simulink model "bus_roadtest_v3"  (R2018a)
settings: Solver=ode3  StartTime=0.0  StopTime=inf  FixedStep=0.01  RelTol=1e-3  EnableMultiTasking=on
PostLoadFcn:
  | , if any(exist('dsrtsu_mdlpostloadfcn', 'file') == [2, 3, 6]), try dsrtsu_mdlpostloadfcn('Execute', bdroot); catch fprintf('Error in PostLoadFcn (dsrtsu_mdlpostloadfcn) for model "%s":\n %s\n', bdroot, lasterr); end, end,
InitFcn:
  | bus_roadtest_v3_initial
values from neighbouring files (symbols this model uses):
  ay_max = 2    [Ini.m]
  delta_t = 0.01    [Ini.m]
  end_left_pass = 1    [Ini.m]
  end_right_pass = 0    [Ini.m]
  finish_node_id = length(Map_data(:,1))    [Ini.m]
  forward_length = 15    [Ini.m]
  gamma = sqrt(N_xaug+lambda)    [bus_roadtest_v3_initial.m]
  k_safe = 1    [Ini.m]
  nodes = nodes(1:index_node,:)    [Ini.m]
  rmin = 10    [Ini.m]
  segments = zeros(length(xy_ends_Pos(:,1)),3)    [Ini.m]
  start_node_id = 1    [Ini.m]
  Ts = 0.01    [bus_roadtest_v3_initial.m]
  Veh_CG = [0.5, 0.2]    [Ini.m]
  Veh_size = [1.99986,6.09558]    [Ini.m]
  vmax = 6    [Ini.m]
  weight = [weight_0,weight_0_cov,weight_i]    [bus_roadtest_v3_initial.m]
undefined symbols (not defined in the file or in its folder): Brake_table, DiscIntNeverNeededParam, Map_data, R, REF_GPS_RFS, Steer_gain_table, T
libraries: rtican x71, simulink x26, rti1401lib_adc_type4 x8, rti1401lib_dio_type4 x1
(part 17 of 18)

== matlab function bus_roadtest_v3/Target_planner/DynamicPathPlanning ==
  data: Path_flag input; Static_Path_0 input size=size(Map_data); Path_final output; XP_final output; YP_final output; Forward_Static_Path_id input size=length(nodes(:,1)); End_x input; End_y input; Vehicle_state input; seg_Curvature input; path_length input; end_right_pass input; end_left_pass input; Veh_CG input; Veh_size input; OB_num input; OBXY input; rmin input; Veh_Velocity input; delta_t input; ay_max input; vmax input; k_safe input; w_off input; LastPath_in input; v_final output; end_point_final output; end_curvature output; TargetXY output; Vehicle_Target_x output; Vehicle_Target_y output; vehicle_boundingbox_x output; vehicle_boundingbox_y output; J_out output; Jminind output; J_finalind output; L_path_final output; collision_check output
function [Path_final,XP_final,YP_final,v_final,end_point_final,end_curvature,TargetXY,Vehicle_Target_x,Vehicle_Target_y,vehicle_boundingbox_x,vehicle_boundingbox_y,J_out,Jminind,J_finalind,L_path_final,collision_check] = DynamicPathPlanning(Path_flag,Static_Path_0,Forward_Static_Path_id,End_x,End_y,Vehicle_state,seg_Curvature,path_length,end_right_pass,end_left_pass,Veh_CG,Veh_size,OB_num,OBXY,rmin,Veh_Velocity,delta_t,ay_max,vmax,k_safe,w_off,LastPath_in)

persistent LastPath
if isempty(LastPath)
    LastPath = zeros(11,2);
else
    LastPath = LastPath_in;
end

x_vehicle = Vehicle_state(1,1); %vehicle global coordinate
y_vehicle = Vehicle_state(2,1);
start_heading = Vehicle_state(3,1);

end_heading_0 = Static_Path_0(Forward_Static_Path_id(end) == Static_Path_0(:,1),8)*pi/180;
end_curvature_0 = Static_Path_0(Forward_Static_Path_id(end) == Static_Path_0(:,1),14);
end_seg_LaneWidth_0 = Static_Path_0(Forward_Static_Path_id(end) == Static_Path_0(:,1),11);
end_heading = end_heading_0(1);
end_curvature = end_curvature_0(1);
end_seg_LaneWidth = end_seg_LaneWidth_0(1);

delta_offset = end_seg_LaneWidth/4;
offset_1 = delta_offset*1;
offset_2 = delta_offset*2;
offset_3 = delta_offset*3;
offset_4 = delta_offset*4;
offset_5 = delta_offset*5;
offset_6 = delta_offset*6;
offset = [offset_6 offset_5 offset_4 offset_3 offset_2 offset_1 0 offset_1 offset_2 offset_3 offset_4 offset_5 offset_6];

x_endpoint1 = End_x + offset_6*cos(end_heading+pi/2);
y_endpoint1 = End_y + offset_6*sin(end_heading+pi/2);
x_endpoint2 = End_x + offset_5*cos(end_heading+pi/2);
y_endpoint2 = End_y + offset_5*sin(end_heading+pi/2);
x_endpoint3 = End_x + offset_4*cos(end_heading+pi/2);
y_endpoint3 = End_y + offset_4*sin(end_heading+pi/2);
x_endpoint4 = End_x + offset_3*cos(end_heading+pi/2);
y_endpoint4 = End_y + offset_3*sin(end_heading+pi/2);
x_endpoint5 = End_x + offset_2*cos(end_heading+pi/2);
y_endpoint5 = End_y + offset_2*sin(end_heading+pi/2);
x_endpoint6 = End_x + offset_1*cos(end_heading+pi/2);
y_endpoint6 = End_y + offset_1*sin(end_heading+pi/2);
x_endpoint7 = End_x;
y_endpoint7 = End_y;
x_endpoint8 = End_x + offset_1*cos(end_heading-pi/2);
y_endpoint8 = End_y + offset_1*sin(end_heading-pi/2);
x_endpoint9 = End_x + offset_2*cos(end_heading-pi/2);
y_endpoint9 = End_y + offset_2*sin(end_heading-pi/2);
x_endpoint10 = End_x + offset_3*cos(end_heading-pi/2);
y_endpoint10 = End_y + offset_3*sin(end_heading-pi/2);
x_endpoint11 = End_x + offset_4*cos(end_heading-pi/2);
y_endpoint11 = End_y + offset_4*sin(end_heading-pi/2);
x_endpoint12 = End_x + offset_5*cos(end_heading-pi/2);
y_endpoint12 = End_y + offset_5*sin(end_heading-pi/2);
x_endpoint13 = End_x + offset_6*cos(end_heading-pi/2);
y_endpoint13 = End_y + offset_6*sin(end_heading-pi/2);

%% Candidate paths generation
[X1,Y1,XP1,YP1,K1,K_11,L_path1] = G2splines(x_vehicle,y_vehicle,start_heading,seg_Curvature,x_endpoint1,y_endpoint1,end_heading,end_curvature,path_length);
[X2,Y2,XP2,YP2,K2,K_12,L_path2] = G2splines(x_vehicle,y_vehicle,start_heading,seg_Curvature,x_endpoint2,y_endpoint2,end_heading,end_curvature,path_length);
[X3,Y3,XP3,YP3,K3,K_13,L_path3] = G2splines(x_vehicle,y_vehicle,start_heading,seg_Curvature,x_endpoint3,y_endpoint3,end_heading,end_curvature,path_length);
[X4,Y4,XP4,YP4,K4,K_14,L_path4] = G2splines(x_vehicle,y_vehicle,start_heading,seg_Curvature,x_endpoint4,y_endpoint4,end_heading,end_curvature,path_length);
[X5,Y5,XP5,YP5,K5,K_15,L_path5] = G2splines(x_vehicle,y_vehicle,start_heading,seg_Curvature,x_endpoint5,y_endpoint5,end_heading,end_curvature,path_length);
[X6,Y6,XP6,YP6,K6,K_16,L_path6] = G2splines(x_vehicle,y_vehicle,start_heading,seg_Curvature,x_endpoint6,y_endpoint6,end_heading,end_curvature,path_length);
[X7,Y7,XP7,YP7,K7,K_17,L_path7] = G2splines(x_vehicle,y_vehicle,start_heading,seg_Curvature,x_endpoint7,y_endpoint7,end_heading,end_curvature,path_length);
[X8,Y8,XP8,YP8,K8,K_18,L_path8] = G2splines(x_vehicle,y_vehicle,start_heading,seg_Curvature,x_endpoint8,y_endpoint8,end_heading,end_curvature,path_length);
[X9,Y9,XP9,YP9,K9,K_19,L_path9] = G2splines(x_vehicle,y_vehicle,start_heading,seg_Curvature,x_endpoint9,y_endpoint9,end_heading,end_curvature,path_length);
[X10,Y10,XP10,YP10,K10,K_110,L_path10] = G2splines(x_vehicle,y_vehicle,start_heading,seg_Curvature,x_endpoint10,y_endpoint10,end_heading,end_curvature,path_length);
[X11,Y11,XP11,YP11,K11,K_111,L_path11] = G2splines(x_vehicle,y_vehicle,start_heading,seg_Curvature,x_endpoint11,y_endpoint11,end_heading,end_curvature,path_length);
[X12,Y12,XP12,YP12,K12,K_112,L_path12] = G2splines(x_vehicle,y_vehicle,start_heading,seg_Curvature,x_endpoint12,y_endpoint12,end_heading,end_curvature,path_length);
[X13,Y13,XP13,YP13,K13,K_113,L_path13] = G2splines(x_vehicle,y_vehicle,start_heading,seg_Curvature,x_endpoint13,y_endpoint13,end_heading,end_curvature,path_length);

X = [X1 X2 X3 X4 X5 X6 X7 X8 X9 X10 X11 X12 X13];
Y = [Y1 Y2 Y3 Y4 Y5 Y6 Y7 Y8 Y9 Y10 Y11 Y12 Y13];
XP = [XP1 XP2 XP3 XP4 XP5 XP6 XP7 XP8 XP9 XP10 XP11 XP12 XP13];
YP = [YP1 YP2 YP3 YP4 YP5 YP6 YP7 YP8 YP9 YP10 YP11 YP12 YP13];
K = [K1 K2 K3 K4 K5 K6 K7 K8 K9 K10 K11 K12 K13];
K_1 = [K_11 K_12 K_13 K_14 K_15 K_16 K_17 K_18 K_19 K_110 K_111 K_112 K_113];
L_path = [L_path1 L_path2 L_path3 L_path4 L_path5 L_path6 L_path7 L_path8 L_path9 L_path10 L_path11 L_path12 L_path13];
xy_end_point = [x_endpoint1,x_endpoint2,x_endpoint3,x_endpoint4,x_endpoint5,x_endpoint6,x_endpoint7,x_endpoint8,x_endpoint9,x_endpoint10,x_endpoint11,x_endpoint12,x_endpoint13;y_endpoint1,y_endpoint2,y_endpoint3,y_endpoint4,y_endpoint5,y_endpoint6,y_endpoint7,y_endpoint8,y_endpoint9,y_endpoint10,y_endpoint11,y_endpoint12,y_endpoint13];

%% Collision check
Path_col = zeros(4,length(X(1,:))); %[Collision T/F ; Path collision ind ; OB num ; Lane collision T/F]
% Lane collision check
if end_right_pass == 0
    Path_col(4,9:13) = 1;
end
if end_left_pass == 0
    Path_col(4,1:5) = 1;
end

% Obstacle collision check
% Obstacle enlarge
OBXY_EL = OBXY;
OB_enlargescale = 0.3;
OB_enlargescale_behind = 0.3;
for m = 1 : OB_num
    OBXY_m = OBXY(2*m-1:2*m,1:4);
    OBXY_EL(2*m-1:2*m,1) = [OBXY_m(1,1) + (OBXY_m(1,1)-OBXY_m(1,2))*OB_enlargescale + (OBXY_m(1,1)-OBXY_m(1,4))*OB_enlargescale ; OBXY_m(2,1) + (OBXY_m(2,1)-OBXY_m(2,2))*OB_enlargescale + (OBXY_m(2,1)-OBXY_m(2,4))*OB_enlargescale];
    OBXY_EL(2*m-1:2*m,2) = [OBXY_m(1,2) + (OBXY_m(1,2)-OBXY_m(1,1))*OB_enlargescale + (OBXY_m(1,2)-OBXY_m(1,3))*OB_enlargescale ; OBXY_m(2,2) + (OBXY_m(2,2)-OBXY_m(2,1))*OB_enlargescale + (OBXY_m(2,2)-OBXY_m(2,3))*OB_enlargescale];
    OBXY_EL(2*m-1:2*m,3) = [OBXY_m(1,3) + (OBXY_m(1,3)-OBXY_m(1,4))*OB_enlargescale + (OBXY_m(1,3)-OBXY_m(1,2))*OB_enlargescale_behind ; OBXY_m(2,3) + (OBXY_m(2,3)-OBXY_m(2,4))*OB_enlargescale + (OBXY_m(2,3)-OBXY_m(2,2))*OB_enlargescale_behind];
    OBXY_EL(2*m-1:2*m,4) = [OBXY_m(1,4) + (OBXY_m(1,4)-OBXY_m(1,3))*OB_enlargescale + (OBXY_m(1,4)-OBXY_m(1,1))*OB_enlargescale_behind ; OBXY_m(2,4) + (OBXY_m(2,4)-OBXY_m(2,3))*OB_enlargescale + (OBXY_m(2,4)-OBXY_m(2,1))*OB_enlargescale_behind];
end
% 計算每條線的每個sample點的單位向量及法向量
X_1 = X(1:end-1,:);
X_2 = X(2:end,:);
X_diff_0 = X_2 - X_1;
X_diff = [X_diff_0(:,:);X_diff_0(end,:)];
Y_1 = Y(1:end-1,:);
Y_2 = Y(2:end,:);
Y_diff_0 = Y_2 - Y_1;
Y_diff = [Y_diff_0(:,:);Y_diff_0(end,:)];
XY_difflen = (X_diff.^2 + Y_diff.^2).^0.5;
X_UV = X_diff./XY_difflen; %X方向單位向量(Unit Vector)
Y_UV = Y_diff./XY_difflen; %Y方向單位向量(Unit Vector)
X_NV = -Y_UV; %X方向單位法向量(Normal Vector)
Y_NV = X_UV; %Y方向單位法向量(Normal Vector)
% 計算veh四個角位置
Path_vehFLX = X + Veh_CG(1)*Veh_size(1).*X_NV + Veh_CG(2)*Veh_size(2).*X_UV;
Path_vehFLY = Y + Veh_CG(1)*Veh_size(1).*Y_NV + Veh_CG(2)*Veh_size(2).*Y_UV;
Path_vehFRX = X - (1-Veh_CG(1))*Veh_size(1).*X_NV + Veh_CG(2)*Veh_size(2).*X_UV;
Path_vehFRY = Y - (1-Veh_CG(1))*Veh_size(1).*Y_NV + Veh_CG(2)*Veh_size(2).*Y_UV;
Path_vehRLX = X + Veh_CG(1)*Veh_size(1).*X_NV - (1-Veh_CG(2))*Veh_size(2).*X_UV;
Path_vehRLY = Y + Veh_CG(1)*Veh_size(1).*Y_NV - (1-Veh_CG(2))*Veh_size(2).*Y_UV;
Path_vehRRX = X - (1-Veh_CG(1))*Veh_size(1).*X_NV - (1-Veh_CG(2))*Veh_size(2).*X_UV;
Path_vehRRY = Y - (1-Veh_CG(1))*Veh_size(1).*Y_NV - (1-Veh_CG(2))*Veh_size(2).*Y_UV;
% project to normal vector
for i = 1 : length(Path_vehFLX(1,:))
    Path_col(1,i) = 0;
    if Path_col(4,i) == 1
        continue;
    else
        for j = 1 : length(Path_vehFLX(:,1))
            Path_vehvol = [Path_vehFLX(j,i),Path_vehFRX(j,i),Path_vehRLX(j,i),Path_vehRRX(j,i);Path_vehFLY(j,i),Path_vehFRY(j,i),Path_vehRLY(j,i),Path_vehRRY(j,i)];
            for k = 1 : OB_num
                OBXY_k = OBXY_EL(2*k-1:2*k,1:4);
                % obstcale normal vector
                OBnormal1 = [-(OBXY_k(2,2)-OBXY_k(2,1)),(OBXY_k(1,2)-OBXY_k(1,1))]./sqrt((OBXY_k(1,2)-OBXY_k(1,1))^2 + (OBXY_k(1,2)-OBXY_k(1,1))^2);
                OBnormal2 = [-(OBXY_k(2,3)-OBXY_k(2,2)),(OBXY_k(1,3)-OBXY_k(1,2))]./sqrt((OBXY_k(2,3)-OBXY_k(2,2))^2 + (OBXY_k(1,3)-OBXY_k(1,2))^2);
                proj_veh = [OBnormal1;OBnormal2;[X_UV(j,i),Y_UV(j,i)];[X_NV(j,i),Y_NV(j,i)]] * Path_vehvol;
                proj_ob = [OBnormal1;OBnormal2;[X_UV(j,i),Y_UV(j,i)];[X_NV(j,i),Y_NV(j,i)]] * OBXY_k;
                minmax_veh = [min(proj_veh,[],2),max(proj_veh,[],2)];
                minmax_obj = [min(proj_ob,[],2),max(proj_ob,[],2)];

                % check if vehicle collide with specify object at the chosen point
                for r = 1:4
                    if (minmax_veh(r,1)>minmax_obj(r,2) || minmax_veh(r,2)<minmax_obj(r,1))
                        Path_col(1,i) = 0;
                        break;      % ends SAT with a object
                    end
                    Path_col(1,i) = 1;
                end
                % Collision happens and ends the object checking process
                if Path_col(1,i) == 1
                    Path_col(3,i) = k;
                    break;         % ends all object checking
                end
            end
            % Collision happens and ends the point checking process
            if Path_col(1,i) == 1
                Path_col(2,i) = j;
                break;          % ends point checking
            end
        end
    end
end
% Gaussian concolution
Cobs_0 = Path_col(1,:);
Cobs = Cobs_0;
sigma = std(Cobs_0(1,:));
delta_q = 1;
Path_index = 1:1:length(Cobs_0(1,:));
if sigma ~= 0
    for i = 1 : length(Cobs_0(1,:))
        Path_index_i = i*ones(size(Path_index));
        Path_index_diff = Path_index_i - Path_index;
        g = exp(-(delta_q.*Path_index_diff).^2./(2*sigma^2))./(sqrt(2*pi)*sigma);
        Cobs(1,i) = sum(Cobs_0(1,:).*g);
        if i == 1 && Cobs_0(1,1) == 1
            Cobs(1,i) = Cobs(1,i) + exp(-(delta_q.*1).^2./(2*sigma^2))./(sqrt(2*pi)*sigma);
        elseif i == length(Cobs_0(1,:)) && Cobs_0(1,end) == 1
            Cobs(1,i) = Cobs(1,i) + exp(-(delta_q.*1).^2./(2*sigma^2))./(sqrt(2*pi)*sigma);
        else
            Cobs(1,i) = Cobs(1,i);
        end
    end
    if max(Cobs(1,:)) ~= 1
        Cobs(1,:) = Cobs(1,:)./max(Cobs(1,:));
    end
end
% Cobs1 = Cobs;
% if sigma ~= 0
%     Cobs1(1,:) = imgaussfilt(Path_col(1,:),sigma); %matlab內建gaussian concolution
% end
Clane_0 = Path_col(4,:);
Clane = Clane_0;
sigma = std(Clane_0(1,:));
delta_q = 1;
Path_index = 1:1:length(Clane_0(1,:));
if sigma ~= 0
    for i = 1 : length(Clane_0(1,:))
        Path_index_i = i*ones(size(Path_index));
        Path_index_diff = Path_index_i - Path_index;
        g = exp(-(delta_q.*Path_index_diff).^2./(2*sigma^2))./(sqrt(2*pi)*sigma);
        Clane(1,i) = sum(Clane_0(1,:).*g);
        if i == 1 && Clane_0(1,1) == 1
            Clane(1,i) = Clane(1,i) + exp(-(delta_q.*1).^2./(2*sigma^2))./(sqrt(2*pi)*sigma);
        elseif i == length(Clane_0(1,:)) && Clane_0(1,end) == 1
            Clane(1,i) = Clane(1,i) + exp(-(delta_q.*1).^2./(2*sigma^2))./(sqrt(2*pi)*sigma);
        else
            Clane(1,i) = Clane(1,i);
        end
    end
    if max(Clane(1,:)) ~= 1
        Clane(1,:) = Clane(1,:)./max(Clane(1,:));
    end
end
%% Consistency
Cc_0 = zeros(1,length(X(1,:)));
% current vehicle postion to last path
[~,Lastpath_si] = min(sqrt((LastPath(:,1) - x_vehicle).^2 + (LastPath(:,2) - y_vehicle).^2));
LastPath_overlap = LastPath(Lastpath_si:end,:);

for k = 1 : length(X(1,:))
    % last end point to current paths
    [~,Pathk_ei] = min(sqrt((X(:,k) - LastPath(end,1)).^2 + (Y(:,k) - LastPath(end,2)).^2));
    Path_overlap = [X(1:Pathk_ei,k) Y(1:Pathk_ei,k)];
%     if length(LastPath_overlap(:,1)) >= length(Path_overlap(:,1))
%         Path_diff = length(LastPath_overlap(:,1)) - length(Path_overlap(:,1));
%         Path_dis = sqrt(sum(LastPath_overlap(1+Path_diff:end,:)-Path_overlap).^2);
%     else
%         Path_diff = length(Path_overlap(:,1)) - length(LastPath_overlap(:,1));
%         Path_dis = sqrt(sum(LastPath_overlap-Path_overlap(1+Path_diff:end,:)).^2);
%     end
    if length(LastPath_overlap(:,1)) >= length(Path_overlap(:,1))
        Path_diff = length(LastPath_overlap(:,1)) - length(Path_overlap(:,1));
%         Path_dis_xy = LastPath_overlap(1+Path_diff:end,:)-Path_overlap;
%         Path_dis = sqrt(Path_dis_xy(:,1).*Path_dis_xy(:,1) + Path_dis_xy(:,2).*Path_dis_xy(:,2));
        Path_dis_xy = (LastPath_overlap(1+Path_diff:end,:)-Path_overlap).^2;
        Path_dis = sqrt(sum(Path_dis_xy'));
        Path_dis = Path_dis';
    else
        Path_diff = length(Path_overlap(:,1)) - length(LastPath_overlap(:,1));
        Path_dis_xy = (LastPath_overlap(1:end,1:2) - Path_overlap(1:end-Path_diff,:)).^2;
        Path_dis = sqrt(sum(Path_dis_xy'));
        Path_dis = Path_dis';
    end
    if mod(length(Path_dis),2) == 0
        cons_simCoeff = 4*ones(1,length(Path_dis)-1);
    else
        cons_simCoeff = 4*ones(1,length(Path_dis));
    end
    cons_simCoeff([1,length(cons_simCoeff)]) = 1;
    cons_simCoeff(3:2:length(cons_simCoeff)-2) = 2;
    
    bframe_delta = L_path(k)/length(X(:,k));
    cons_overlapL = L_path(k)*length(Path_dis)/length(X(:,k));
    Path_sumdis = bframe_delta*(cons_simCoeff*Path_dis(1:length(cons_simCoeff))')/3;
    Cc_0(1,k) = Path_sumdis/cons_overlapL;
end

%% Cost function
% weighting
W = [0.5 1 1 w_off 30 10 30];
%   [ L   k  k_1 off obs c lane]

Cl = L_path./path_length;
Ck = (max(abs(K)).*rmin)./max(max(abs(K)).*rmin);
Ck_1 = (max(abs(K_1)).*rmin)./max(max(abs(K_1)).*rmin);
Coff = offset/max(offset);
Cobss = Cobs(1,:);%Path_col(1,:);%f*exp((-1/lamda).*d) + P;
if max(Cc_0) == 0
    Cc = Cc_0;
else
    Cc = Cc_0/max(Cc_0);
end
Clanes = Clane(1,:);%Path_col(1,:);%f*exp((-1/lamda).*d) + P;

% cost function
J = W(1).*Cl + W(2).*Ck + W(3).*Ck_1 + W(4).*Coff + W(5).*Cobss + W(6).*Cc + W(7).*Clanes;
[Jmin,Jminind] = min(J);

if Path_flag == 1
    J_finalind = Jminind;
else
    J_finalind = 7;
end

X_final = X(:,J_finalind);
Y_final = Y(:,J_finalind);
Path_final = [X_final,Y_final];
end_point_final = [xy_end_point(:,J_finalind);end_heading];
J_out = J';

%% Velocity decision
k_vehicle_max = 1/rmin;
if max(abs(K(J_finalind))) > k_vehicle_max
    k_max = k_vehicle_max;
else
    k_max = max(abs(K(J_finalind)));
end
v_k = sqrt(ay_max/k_max);
v_safe = (1-k_safe*Cobs(J_finalind)^2)*v_k;
if v_safe > vmax
    v_final = vmax; %(m/s)
else
    v_final = v_safe; %(m/s)
end

L_path_final = L_path(J_finalind);

%% Next Step Position
XP_final = XP(:,J_finalind);
YP_final = YP(:,J_finalind);
u_final_Target = (Veh_Velocity*1+3)/L_path(J_finalind);
x_target = XP_final(1) + XP_final(2)*u_final_Target + XP_final(3)*u_final_Target^2 + XP_final(4)*u_final_Target^3 + XP_final(5)*u_final_Target^4 + XP_final(6)*u_final_Target^5;
y_target = YP_final(1) + YP_final(2)*u_final_Target + YP_final(3)*u_final_Target^2 + YP_final(4)*u_final_Target^3 + YP_final(5)*u_final_Target^4 + YP_final(6)*u_final_Target^5;
TargetXY = [x_target;y_target];
vehicle_boundingbox_x = [Path_vehFLX(1,7);Path_vehFRX(1,7);Path_vehRRX(1,7);Path_vehRLX(1,7)];
vehicle_boundingbox_y = [Path_vehFLY(1,7);Path_vehFRY(1,7);Path_vehRRY(1,7);Path_vehRLY(1,7)];
%% vehicle target x y
heading = Vehicle_state(3,1);
rotate_ang = -heading;
Vehicle_Target = [cos(rotate_ang),-sin(rotate_ang);sin(rotate_ang),cos(rotate_ang)]*[x_target-x_vehicle;y_target-y_vehicle];
Vehicle_Target_x = Vehicle_Target(1);
Vehicle_Target_y = Vehicle_Target(2);

%%
collision_check = Cobs_0(J_finalind);
%% Function
function [X,Y,XP,YP,K,K_1,L_path] = G2splines(xa,ya,thetaa,ka,xb,yb,thetab,kb,path_length)
n1 = path_length; %optimization
n2 = n1;
n3 = 0; %越大切越大
n4 = -n3;

% n1 = path_length; %optimization
% n2 = n1;
% n3 = 50; %越大切越大
% n4 = -n3;

% n1 = path_length/3; %optimization
% n2 = n1;
% n3 = 50; %optimization
% n4 = -n3;

x0 = xa;
x1 = n1*cos(thetaa);
x2 = 0.5*(n3*cos(thetaa)-(n1^2)*ka*sin(thetaa));
x3 = 10*(xb-xa)-(6*n1+1.5*n3).*cos(thetaa)-(4*n2-0.5*n4).*cos(thetab)+1.5*(n1^2)*ka.*sin(thetaa)-0.5*(n2^2)*kb.*sin(thetab);
x4 = -15*(xb-xa)+(8*n1+1.5*n3).*cos(thetaa)+(7*n2-n4).*cos(thetab)-1.5*(n1^2)*ka.*sin(thetaa)+(n2^2)*kb.*sin(thetab);
x5 = 6*(xb-xa)-(3*n1+0.5*n3).*cos(thetaa)-(3*n2-0.5*n4).*cos(thetab)+0.5*(n1^2)*ka.*sin(thetaa)-0.5*(n2^2)*kb.*sin(thetab);
XP = [x0;x1;x2;x3;x4;x5];

y0 = ya;
y1 = n1*sin(thetaa);
y2 = 0.5*(n3*sin(thetaa)+(n1^2)*ka*cos(thetaa));
y3 = 10*(yb-ya)-(6*n1+1.5*n3).*sin(thetaa)-(4*n2-0.5*n4).*sin(thetab)-1.5*(n1^2)*ka.*cos(thetaa)+0.5*(n2^2)*kb.*cos(thetab);
y4 = -15*(yb-ya)+(8*n1+1.5*n3).*sin(thetaa)+(7*n2-n4).*sin(thetab)+1.5*(n1^2)*ka.*cos(thetaa)-(n2^2)*kb.*cos(thetab);
y5 = 6*(yb-ya)-(3*n1+0.5*n3).*sin(thetaa)-(3*n2-0.5*n4).*sin(thetab)-0.5.*(n1^2)*ka*cos(thetaa)+0.5.*(n2^2)*kb.*cos(thetab);
YP = [y0;y1;y2;y3;y4;y5];

u = 0 : 0.1 : 1;
u = u';
X = x0 + x1.*u + x2.*u.^2 + x3.*u.^3 + x4.*u.^4 + x5.*u.^5;
Y = y0 + y1.*u + y2.*u.^2 + y3.*u.^3 + y4.*u.^4 + y5.*u.^5;
X_1 = x1 + x2*2*u + x3*3*u.^2 + x4*4*u.^3 + x5*5*u.^4;
X_2 = x2*2 + x3*6*u + x4*12*u.^2 + x5*20*u.^3;
X_3 = x3*6 + x4*24*u + x5*60*u.^2;
Y_1 = y1 + y2*2*u + y3*3*u.^2 + y4*4*u.^3 + y5*5*u.^4;
Y_2 = y2*2 + y3*6*u + y4*12*u.^2 + y5*20*u.^3;
Y_3 = y3*6 + y4*24*u + y5*60*u.^2;
K = (X_1.*Y_2-X_2.*Y_1)./((X_1.^2+Y_1.^2).^1.5);
K_1 = ((X_1.^2+Y_1.^2).^1.5.*(X_2.*Y_2+X_1.*Y_3-X_3.*Y_1-X_2.*Y_2)-1.5.*(X_1.*Y_2-X_2.*Y_1).*(2.*X_1.*X_2+2.*Y_1.*Y_2).*((X_1.^2+Y_1.^2).^0.5))./((X_1.^2+Y_1.^2).^3);

% syms t
% XX_1 = x1 + x2*2*t + x3*3*t^2 + x4*4*t^3 + x5*5*t^4;
% YY_1 = y1 + y2*2*t + y3*3*t^2 + y4*4*t^3 + y5*5*t^4;
% f = (XX_1.^2+YY_1.^2).^0.5;
% L_path = double(int(f,t,0,1));
L_path = path_length;

== matlab function bus_roadtest_v3/Speed_profile/Auto & Check/Auto_start ==
  settings: updateMethod=DISCRETE
  data: Stop_Check input; Obj_detect input; AutoStart output; Emergency_stop input; AEB_count output; Drive_stop input; Drive_start input; AEBStatic output; AEBOn output; Static_flag input
function [AutoStart, AEB_count, AEBStatic, AEBOn] = fcn(Stop_Check, Obj_detect,Emergency_stop,Drive_stop,Drive_start, Static_flag)
persistent AEB_on counting AEB_static
if isempty(AEB_on)
    AEB_on = 0;
    counting = 0;
    AEB_static = 1;
end 
AutoStart = 0;

% if Obj_detect ==1 && Idle_flag ==0
if Obj_detect ==1
    AEB_on = 1;
end
if AEB_on==1 && Obj_detect==0 && Static_flag==1
    counting = counting+1;
elseif AEB_on==1 && Obj_detect==1
    counting = 0;
end
if counting>300 
    AEB_on = 0;
    counting = 0;
    AutoStart = 1;
end


% AEB_static will overwrite AutoStart
if Emergency_stop ==1 || Drive_stop ==1 ||  Stop_Check==1
    AEB_static = 1;
elseif Drive_start ==1
    AEB_static = 0;
    AEB_on = 0;
    counting = 0;
end
if AEB_static == 1
    AutoStart = 0;
end


% Output state
AEB_count = counting;
AEBStatic = AEB_static;
AEBOn = AEB_on;

== matlab function bus_roadtest_v3/Target_planner/DynamicPathPlanning1 ==
  data: Static_Path_0 input size=size(Map_data); Path_final output; XP_final output; YP_final output; Forward_Static_Path_id input size=length(nodes(:,1)); End_x input; End_y input; Jminind input; x_vehicle input; y_vehicle input; start_heading input; seg_Curvature input; path_length input; Veh_CG input; Veh_size input; OB_num input; OBXY input; collision_check output
function [Path_final,XP_final,YP_final,collision_check] = DynamicPathPlanning(Static_Path_0,Forward_Static_Path_id,End_x,End_y,Jminind,x_vehicle,y_vehicle,start_heading,seg_Curvature,path_length,Veh_CG,Veh_size,OB_num,OBXY)

% x_vehicle = Vehicle_state(1,1); %vehicle global coordinate
% y_vehicle = Vehicle_state(2,1);
% start_heading = Vehicle_state(3,1);

end_heading_0 = Static_Path_0(Forward_Static_Path_id(end) == Static_Path_0(:,1),8)*pi/180;
end_curvature_0 = Static_Path_0(Forward_Static_Path_id(end) == Static_Path_0(:,1),14);
end_seg_LaneWidth_0 = Static_Path_0(Forward_Static_Path_id(end) == Static_Path_0(:,1),11);
end_heading = end_heading_0(1);
end_curvature = end_curvature_0(1);
end_seg_LaneWidth = end_seg_LaneWidth_0(1);

delta_offset = end_seg_LaneWidth/4;
offset_1 = delta_offset*1;
offset_2 = delta_offset*2;
offset_3 = delta_offset*3;
offset_4 = delta_offset*4;
offset_5 = delta_offset*5;
offset_6 = delta_offset*6;
offset = [offset_6 offset_5 offset_4 offset_3 offset_2 offset_1 0 offset_1 offset_2 offset_3 offset_4 offset_5 offset_6];

offset_final = offset(Jminind);

if Jminind < 8
    x_endpoint = End_x + offset_final*cos(end_heading+pi/2);
    y_endpoint = End_y + offset_final*sin(end_heading+pi/2);
else
    x_endpoint = End_x + offset_final*cos(end_heading-pi/2);
    y_endpoint = End_y + offset_final*sin(end_heading-pi/2);
end

%% Candidate paths generation
[X_final,Y_final,XP_final,YP_final,K2,K_12,L_path2] = G2splines(x_vehicle,y_vehicle,start_heading,seg_Curvature,x_endpoint,y_endpoint,end_heading,end_curvature,path_length);
Path_final = [X_final,Y_final];

%% Collision check
Path_col = zeros(3,1); %[Collision T/F ; Path collision ind ; OB num ; Lane collision T/F]
% Obstacle collision check
% 計算每條線的每個sample點的單位向量及法向量
X_1 = X_final(1:end-1);
X_2 = X_final(2:end);
X_diff_0 = X_2 - X_1;
X_diff = [X_diff_0(:,:);X_diff_0(end,:)];
Y_1 = Y_final(1:end-1);
Y_2 = Y_final(2:end);
Y_diff_0 = Y_2 - Y_1;
Y_diff = [Y_diff_0(:,:);Y_diff_0(end,:)];
XY_difflen = (X_diff.^2 + Y_diff.^2).^0.5;
X_UV = X_diff./XY_difflen; %X方向單位向量(Unit Vector)
Y_UV = Y_diff./XY_difflen; %Y方向單位向量(Unit Vector)
X_NV = -Y_UV; %X方向單位法向量(Normal Vector)
Y_NV = X_UV; %Y方向單位法向量(Normal Vector)
% 計算veh四個角位置
Path_vehFLX = X_final + Veh_CG(1)*Veh_size(1).*X_NV + Veh_CG(2)*Veh_size(2).*X_UV;
Path_vehFLY = Y_final + Veh_CG(1)*Veh_size(1).*Y_NV + Veh_CG(2)*Veh_size(2).*Y_UV;
Path_vehFRX = X_final - (1-Veh_CG(1))*Veh_size(1).*X_NV + Veh_CG(2)*Veh_size(2).*X_UV;
Path_vehFRY = Y_final - (1-Veh_CG(1))*Veh_size(1).*Y_NV + Veh_CG(2)*Veh_size(2).*Y_UV;
Path_vehRLX = X_final + Veh_CG(1)*Veh_size(1).*X_NV - (1-Veh_CG(2))*Veh_size(2).*X_UV;
Path_vehRLY = Y_final + Veh_CG(1)*Veh_size(1).*Y_NV - (1-Veh_CG(2))*Veh_size(2).*Y_UV;
Path_vehRRX = X_final - (1-Veh_CG(1))*Veh_size(1).*X_NV - (1-Veh_CG(2))*Veh_size(2).*X_UV;
Path_vehRRY = Y_final - (1-Veh_CG(1))*Veh_size(1).*Y_NV - (1-Veh_CG(2))*Veh_size(2).*Y_UV;
% project to normal vector
Path_col(1) = 0;
for j = 1 : length(Path_vehFLX(:,1))
    Path_vehvol = [Path_vehFLX(j),Path_vehFRX(j),Path_vehRLX(j),Path_vehRRX(j);Path_vehFLY(j),Path_vehFRY(j),Path_vehRLY(j),Path_vehRRY(j)];
    for k = 1 : OB_num
        OBXY_k = OBXY(2*k-1:2*k,1:4);
        % obstcale normal vector
        OBnormal1 = [-(OBXY_k(2,2)-OBXY_k(2,1)),(OBXY_k(1,2)-OBXY_k(1,1))]./sqrt((OBXY_k(1,2)-OBXY_k(1,1))^2 + (OBXY_k(1,2)-OBXY_k(1,1))^2);
        OBnormal2 = [-(OBXY_k(2,3)-OBXY_k(2,2)),(OBXY_k(1,3)-OBXY_k(1,2))]./sqrt((OBXY_k(2,3)-OBXY_k(2,2))^2 + (OBXY_k(1,3)-OBXY_k(1,2))^2);
        proj_veh = [OBnormal1;OBnormal2;[X_UV(j),Y_UV(j)];[X_NV(j),Y_NV(j)]] * Path_vehvol;
        proj_ob = [OBnormal1;OBnormal2;[X_UV(j),Y_UV(j)];[X_NV(j),Y_NV(j)]] * OBXY_k;
        minmax_veh = [min(proj_veh,[],2),max(proj_veh,[],2)];
        minmax_obj = [min(proj_ob,[],2),max(proj_ob,[],2)];

        % check if vehicle collide with specify object at the chosen point
        for r = 1:4
            if (minmax_veh(r,1)>minmax_obj(r,2) || minmax_veh(r,2)<minmax_obj(r,1))
                Path_col(1) = 0;
                break;      % ends SAT with a object
            end
            Path_col(1) = 1;
        end
        % Collision happens and ends the object checking process
        if Path_col(1) == 1
            Path_col(3) = k;
            break;         % ends all object checking
        end
    end
    % Collision happens and ends the point checking process
    if Path_col(1) == 1
        Path_col(2) = j;
        break;          % ends point checking
    end
end
collision_check = Path_col(1);
%% Function
function [X,Y,XP,YP,K,K_1,L_path] = G2splines(xa,ya,thetaa,ka,xb,yb,thetab,kb,path_length)
n1 = path_length; %optimization
n2 = n1;
n3 = 0; %越大切越大
n4 = -n3;

% n1 = path_length; %optimization
% n2 = n1;
% n3 = 50; %越大切越大
% n4 = -n3;

% n1 = path_length/3; %optimization
% n2 = n1;
% n3 = 50; %optimization
% n4 = -n3;

x0 = xa;
x1 = n1*cos(thetaa);
x2 = 0.5*(n3*cos(thetaa)-(n1^2)*ka*sin(thetaa));
x3 = 10*(xb-xa)-(6*n1+1.5*n3).*cos(thetaa)-(4*n2-0.5*n4).*cos(thetab)+1.5*(n1^2)*ka.*sin(thetaa)-0.5*(n2^2)*kb.*sin(thetab);
x4 = -15*(xb-xa)+(8*n1+1.5*n3).*cos(thetaa)+(7*n2-n4).*cos(thetab)-1.5*(n1^2)*ka.*sin(thetaa)+(n2^2)*kb.*sin(thetab);
x5 = 6*(xb-xa)-(3*n1+0.5*n3).*cos(thetaa)-(3*n2-0.5*n4).*cos(thetab)+0.5*(n1^2)*ka.*sin(thetaa)-0.5*(n2^2)*kb.*sin(thetab);
XP = [x0;x1;x2;x3;x4;x5];

y0 = ya;
y1 = n1*sin(thetaa);
y2 = 0.5*(n3*sin(thetaa)+(n1^2)*ka*cos(thetaa));
y3 = 10*(yb-ya)-(6*n1+1.5*n3).*sin(thetaa)-(4*n2-0.5*n4).*sin(thetab)-1.5*(n1^2)*ka.*cos(thetaa)+0.5*(n2^2)*kb.*cos(thetab);
y4 = -15*(yb-ya)+(8*n1+1.5*n3).*sin(thetaa)+(7*n2-n4).*sin(thetab)+1.5*(n1^2)*ka.*cos(thetaa)-(n2^2)*kb.*cos(thetab);
y5 = 6*(yb-ya)-(3*n1+0.5*n3).*sin(thetaa)-(3*n2-0.5*n4).*sin(thetab)-0.5.*(n1^2)*ka*cos(thetaa)+0.5.*(n2^2)*kb.*cos(thetab);
YP = [y0;y1;y2;y3;y4;y5];

u = 0 : 0.1 : 1;
u = u';
X = x0 + x1.*u + x2.*u.^2 + x3.*u.^3 + x4.*u.^4 + x5.*u.^5;
Y = y0 + y1.*u + y2.*u.^2 + y3.*u.^3 + y4.*u.^4 + y5.*u.^5;
X_1 = x1 + x2*2*u + x3*3*u.^2 + x4*4*u.^3 + x5*5*u.^4;
X_2 = x2*2 + x3*6*u + x4*12*u.^2 + x5*20*u.^3;
X_3 = x3*6 + x4*24*u + x5*60*u.^2;
Y_1 = y1 + y2*2*u + y3*3*u.^2 + y4*4*u.^3 + y5*5*u.^4;
Y_2 = y2*2 + y3*6*u + y4*12*u.^2 + y5*20*u.^3;
Y_3 = y3*6 + y4*24*u + y5*60*u.^2;
K = (X_1.*Y_2-X_2.*Y_1)./((X_1.^2+Y_1.^2).^1.5);
K_1 = ((X_1.^2+Y_1.^2).^1.5.*(X_2.*Y_2+X_1.*Y_3-X_3.*Y_1-X_2.*Y_2)-1.5.*(X_1.*Y_2-X_2.*Y_1).*(2.*X_1.*X_2+2.*Y_1.*Y_2).*((X_1.^2+Y_1.^2).^0.5))./((X_1.^2+Y_1.^2).^3);

% syms t
% XX_1 = x1 + x2*2*t + x3*3*t^2 + x4*4*t^3 + x5*5*t^4;
% YY_1 = y1 + y2*2*t + y3*3*t^2 + y4*4*t^3 + y5*5*t^4;
% f = (XX_1.^2+YY_1.^2).^0.5;
% L_path = double(int(f,t,0,1));
L_path = path_length;

== matlab function bus_roadtest_v3/Flag_management/Fault detection/Fault detection(Control)/SLAM fault detection ==
  data: SLAM_FaultFlag input; y output; SLAM_MM_FaultFlag input
function y = fcn(SLAM_FaultFlag, SLAM_MM_FaultFlag)

y = max(SLAM_FaultFlag, SLAM_MM_FaultFlag);

== matlab function bus_roadtest_v3/Motion_controller/Longitudinal_control/Switching_module/MATLAB Function ==
  data: Speed_cmd input; T_resume output; Speed_bound input; upper_ratio input; lower_ratio input
function T_resume = T_shreshold(Speed_cmd,Speed_bound,upper_ratio,lower_ratio)

if Speed_cmd >= Speed_bound
    T_resume = upper_ratio;
else
    T_resume = lower_ratio + (Speed_cmd/Speed_bound)*(upper_ratio-lower_ratio);
end

== matlab function bus_roadtest_v3/Flag_management/State management/ BusStops ==
  settings: updateMethod=DISCRETE
  data: SLAM_X input; SLAM_Y input; Drive_start input; Stop_range input; BusStop_flag output; Stop_Distance output; Stop_cmd input; Stop_Mission input; Bus_state_forstop input; stop_acc output
function [BusStop_flag, Stop_Distance, stop_acc] = fcn(SLAM_X, SLAM_Y, Drive_start, Stop_range, Stop_cmd, Stop_Mission,Bus_state_forstop)

persistent BusStop_state NO_stop 
if isempty(BusStop_state)
    BusStop_state = 0;
    NO_stop = 0;
end 

% For SAND
% Stop_X = [  165.93, 1000000,    1000000,    1000000,    1000000,    1000000,    1000000,    1000000]; 
% Stop_Y = [  64.86,  1000000,    1000000,    1000000,     1000000,    1000000,    1000000,    1000000];


Stop_X = [  -12.192,    323.597,    600.409,    383.098,    33.200, 1000000, 1000000, 1000000]; 
Stop_Y = [  -114.466,   -282.300,   -194.395,   -45.546,    4.324,  1000000, 1000000, 1000000];
Stop_num = size(Stop_cmd,1);
for i=1:1:Stop_num
    if Stop_cmd(i)==0
        Stop_X(i) = 1000000;
        Stop_Y(i) = 1000000;
    end
end

if Stop_Mission ==99
    Stop_Distance = 1000;
else
    Stop_Distance = sqrt((SLAM_X-Stop_X(Stop_Mission))^2 + (SLAM_Y-Stop_Y(Stop_Mission))^2);
end

%%%%%%%%%%%%%%%%%%%%%%%%%%%%%%%%%%%%%%%%%%%%%%%%%%%%%%%%%%%%%%%%%%%%%%%%%%%
% Prevent Drive_start disable in checking zone
if Stop_Distance<5 && Drive_start==1
    NO_stop = 1;
end
if Stop_Distance>5.5 
    NO_stop = 0;
end

%%%%%%%%%%%%%%%%%%%%%%%%%%%%%%%%%%%%%%%%%%%%%%%%%%%%%%%%%%%%%%%%%%%%%%%%%%%
if Drive_start == 1
    BusStop_state = 0;
end
% Use distance for dicision
if Stop_Distance<Stop_range && Stop_Distance>(Stop_range-1) && NO_stop==0 && Bus_state_forstop==1
    BusStop_state = 1;
end
BusStop_flag = BusStop_state;

%%%%%%%%%%%%%%%%%%%%%%%%%%%%%%%%%%%%%%%%%%%%%%%%%%%%%%%%%%%%%%%%%%%%%%%%%%%

% Stop acc from accelerating in stop_zone
if Stop_Distance<30 && Bus_state_forstop==1 
    stop_acc = 1;
else
    stop_acc = 0;
end

== matlab function bus_roadtest_v3/Flag_management/State management/State_Management2 ==
  settings: updateMethod=DISCRETE
  data: Limit_range input; Zig_zag input; Fault_prime input; Fault_minor input; Idle_flag output; AEB_flag output; Digital_gate input; Static_flag input; Drive_start input; Auto_start input; Drive_stop input; BusStop_flag input; SlowMode_flag output; Emergency_stop input; Obj_detect output
function [Idle_flag, AEB_flag, SlowMode_flag, Obj_detect]= fcn(Limit_range,Zig_zag, Fault_prime, Fault_minor, Digital_gate, Static_flag, Drive_start, Auto_start, Drive_stop, BusStop_flag, Emergency_stop)

persistent Idle_state  AEB_state;
if isempty(Idle_state)
    Idle_state = 1;
    AEB_state = 0;
end 
%%%%%%%%%%%%%%%%%%%%%%%%%%%%%%%%%%%%%%%%%%%%%%%%%%%%%%%%%%%%%%%%%%%%%%%%%%%
%For Driving mode control
%Two buttons Drive_start & Drive_stop
% Only way to invalidate Idle_state, and disable AEB_state

% if (Drive_start == 1 || Auto_start == 1) && Static_flag == 1
if (Drive_start == 1 || Auto_start == 1) 
    Idle_state = 0;
    AEB_state= 0;
end
%%%%%%%%%%%%%%%%%%%%%%%%%%%%%%%%%%%%%%%%%%%%%%%%%%%%%%%%%%%%%%%%%%%%%%%%%%%
if Drive_stop == 1 
    Idle_state = 1;
end
%%%%%%%%%%%%%%%%%%%%%%%%%%%%%%%%%%%%%%%%%%%%%%%%%%%%%%%%%%%%%%%%%%%%%%%%%%%
if BusStop_flag == 1 
    Idle_state = 1;
end
%%%%%%%%%%%%%%%%%%%%%%%%%%%%%%%%%%%%%%%%%%%%%%%%%%%%%%%%%%%%%%%%%%%%%%%%%%%
%Fault Flag checking
if Fault_prime == 1
    Idle_state = 1;
end

%%%%%%%%%%%%%%%%%%%%%%%%%%%%%%%%%%%%%%%%%%%%%%%%%%%%%%%%%%%%%%%%%%%%%%%%%%%
% SlowMode_flag
%%%%%%%%%%%%%%%%%%%%%%%%%%%%%%%%%%%%%%%%%%%%%%%%%%%%%%%%%%%%%%%%%%%%%%%%%%%
if max([Zig_zag, Fault_minor]) ==1
    SlowMode_flag = 1;
else
    SlowMode_flag = 0;
end

%%%%%%%%%%%%%%%%%%%%%%%%%%%%%%%%%%%%%%%%%%%%%%%%%%%%%%%%%%%%%%%%%%%%%%%%%%%
% AEB_state
%%%%%%%%%%%%%%%%%%%%%%%%%%%%%%%%%%%%%%%%%%%%%%%%%%%%%%%%%%%%%%%%%%%%%%%%%%%
if    Emergency_stop == 1
    AEB_state = 1;
    Idle_state = 1;
end
%%%%%%%%%%%%%%%%%%%%%%%%%%%%%%%%%%%%%%%%%%%%%%%%%%%%%%%%%%%%%%%%%%%%%%%%%%%
Obj_detect = 0;
if  Digital_gate<Limit_range % For Demo (modified)
    AEB_state = 1;
    Idle_state = 1;
    Obj_detect = 1;
end
%%%%%%%%%%%%%%%%%%%%%%%%%%%%%%%%%%%%%%%%%%%%%%%%%%%%%%%%%%%%%%%%%%%%%%%%%%% 
Idle_flag = Idle_state;
AEB_flag = AEB_state;

== matlab function bus_roadtest_v3/Flag_management/State management/Map_defined_behavior ==
  data: ROS_near_segID input; Uturn_decel output; ROS_target_segID input; Uturn_gain output; Intersection_decel output; Uphill output; Uturn_gain_val output; Uturn_speed output
function [Uturn_decel,Uturn_gain,Intersection_decel,Uphill,Uturn_gain_val,Uturn_speed]  = Map_defined_behavior(ROS_near_segID,ROS_target_segID)

% ========== Initial parameters ==== %
persistent Gain_Uturn Decel_Uturn Decel_intersection Accel_Uphill
if isempty(Gain_Uturn)
    Gain_Uturn = 0;            % LKC gain should change to U-turn mode if Gain_Uturn == 1
    Decel_Uturn = 0;           % Speed_cmd should change to default speed for U-turn
    Decel_intersection = 0;    % Speed_cmd should change to default speed for passing intersection
    Accel_Uphill = 0;          % Speed_cmd should change to default speed for uphill section
end 

% ========== Map parameters =========%

% Map 1127
% intersection_seg = [24,38 ; 230,240];
% Uturn_seg =[4,19,20 ; 
%            43,60,18 ; 
%            75,84,20 ; 
%            97,108,20 ; 
%            109,126,18 ; 
%            155,165,20 ; 
%            168,180,20 ; 
%            203,215,20 ; 
%            219,232,20 ; 
%            285,297,20];
% Uturn_decel_seg = [4,19,7 ; 
%                    43,60,7 ; 
%                    75,84,7 ; 
%                    97,108,6 ; 
%                    109,126,5 ; 
%                    155,165,5 ; 
%                    168,180,5 ; 
%                    203,215,7 ; 
%                    219,232,10 ; 
%                    285,297,10];
% Uphill_seg = [96,104];

% Map 1127 & Rear axis control
intersection_seg = [24,38 ; 230,240];
Uturn_seg =[4,22,20 ; 
           43,65,20 ; 
           75,89,20 ; 
           97,109,20 ; 
           109,132,20 ; 
           155,168,20 ; 
           168,187,20 ; 
           203,216,20 ; 
           219,238,20 ; 
           285,302,20];
Uturn_decel_seg = [4,19,7 ; 
                   43,60,7 ; 
                   75,84,7 ; 
                   97,108,6 ; 
                   109,126,5 ; 
                   155,165,5 ; 
                   168,180,5 ; 
                   203,215,7 ; 
                   219,232,10 ; 
                   285,297,10];
Uphill_seg = [96,104];


% Map Tainan 0309
% intersection_seg = [2500,3000];
% Uturn_seg =[1,14,20 ; 
%            20,30,20 ; 
%            47,68,20 ; 
%            103,115,20 ; 
%            115,131,20 ; 
%            151,184,20 ; 
%            189,203,20 ; 
%            210,223,20 ; 
%            265,275,20 ; 
%            275,288,20 ;
%            327,341,20];
% Uturn_decel_seg = [1,14,5 ; 
%                    20,30,10 ; 
%                    47,68,10 ; 
%                    103,115,7 ; 
%                    115,131,7 ; 
%                    151,175,7 ; 
% %                    189,203,10 ; 
%                    210,223,7 ; 
%                    265,275,7 ; 
%                    275,288,7 ;
%                    327,341,5];
% Uphill_seg = [2000,3000];

% % Map Tainan 0312 (Bus stop)
% intersection_seg = [2500,3000];
% Uturn_seg =[19,30,30];
% Uturn_decel_seg = [2000,3000,10];
% Uphill_seg = [2000,3000];

% ========== Process ================%

for index_inter = 1:length(intersection_seg(:,1))
    if (ROS_target_segID >= intersection_seg(index_inter,1)) && (ROS_target_segID < intersection_seg(index_inter,2))
        Decel_intersection = 1;
        break;
    end
    Decel_intersection = 0;
end

for index_Uturn = 1:length(Uturn_seg(:,1))
    if (ROS_target_segID >= Uturn_seg(index_Uturn,1)) && (ROS_target_segID < Uturn_seg(index_Uturn,2))
        Gain_Uturn = 1;
        Uturn_gain_val = Uturn_seg(index_Uturn,3);
        break;
    end
    Gain_Uturn = 0;
    Uturn_gain_val = -1;
end

for index_Udecel = 1:length(Uturn_decel_seg(:,1))
    if (ROS_target_segID >= Uturn_decel_seg(index_Udecel,1)) && (ROS_target_segID < Uturn_decel_seg(index_Udecel,2))
        Decel_Uturn = 1;
        Uturn_speed = Uturn_decel_seg(index_Udecel,3);
        break;
    end
    Decel_Uturn = 0;
    Uturn_speed = -1;
end

for index_Uphill = 1:length(Uphill_seg(:,1))
    if (ROS_target_segID >= Uphill_seg(index_Uphill,1)) && (ROS_target_segID < Uphill_seg(index_Uphill,2))
        Accel_Uphill = 1;
        break;
    end
    Accel_Uphill = 0;
end

% ========== Flag output ============%

Uturn_gain = Gain_Uturn;
Uphill = Accel_Uphill;
if Uphill == 1
    Uturn_decel = 0;
    Intersection_decel = 0;
    Uturn_speed = -1;
else
    Uturn_decel = Decel_Uturn;
    Intersection_decel = Decel_intersection;
end

== matlab function bus_roadtest_v3/Flag_management/State management/TrafficLight ==
  settings: updateMethod=DISCRETE
  data: Light_Distance output; Light_flag output; Phase input; Light_acc output; SLAM_X input; SLAM_Y input; SLAM_seg_id_near input; Stop_Distance input; Drive_start input
function [Light_Distance, Light_flag, Light_acc] = fcn(Phase, SLAM_X, SLAM_Y,SLAM_seg_id_near, Stop_Distance, Drive_start)

%Stops & Light position on absolute coordinate
Light_X = [108.93, 118.31, 132.78];
Light_Y = [-9.39,  -20.71, -9.88];
Light_stop = [Light_X(3), Light_Y(3)];

% SAND
% Light_X = [  139.2,    160.79,    150.35,    133.28,    117.01, 136.09, 1000000, 1000000]; 
% Light_Y = [  88.74,   48.89,   19.88,   57.21,    92.42,  -11.87, 1000000, 1000000];
% if SLAM_seg_id_near>=114 && SLAM_seg_id_near<135
%     Light_stop = [Light_X(1), Light_Y(1)];
% elseif SLAM_seg_id_near>=135 && SLAM_seg_id_near<155
%     Light_stop = [Light_X(2), Light_Y(2)];
% elseif SLAM_seg_id_near>=218 && SLAM_seg_id_near<241
%     Light_stop = [Light_X(3), Light_Y(3)];
% elseif SLAM_seg_id_near>=241 && SLAM_seg_id_near<254
%     Light_stop = [Light_X(4), Light_Y(4)];
% elseif SLAM_seg_id_near>=254 && SLAM_seg_id_near<268
%     Light_stop = [Light_X(5), Light_Y(5)];
% elseif SLAM_seg_id_near>=309 && SLAM_seg_id_near<330
%     Light_stop = [Light_X(6), Light_Y(6)];
% else
%     Light_stop = [1000000, 1000000];
% end
% if SLAM_seg_id_near>102 && SLAM_seg_id_near<112
%     Light_stop = [Light_X(1), Light_Y(1)];
% elseif SLAM_seg_id_near>=388 && SLAM_seg_id_near<390
%     Light_stop = [Light_X(2), Light_Y(2)];
% else
%     Light_stop = [1000000, 1000000];
% end

persistent Light_state;
if isempty(Light_state)
    Light_state = 0;
end 

Light_Distance = sqrt((SLAM_X - Light_stop(1))^2 + (SLAM_Y - Light_stop(2))^2);
% 
% if Phase ==1 || Phase ==3 
%     if Speed_fb>=17
%        if Light_Distance<Stop_Dis_High && Light_Distance>(Stop_Dis_High-2)
%             Light_state = 1;
%        end
%     elseif Speed_fb>=13 && Speed_fb<17
%        if Light_Distance<Stop_Dis_Mid && Light_Distance>(Stop_Dis_Mid-2)
%             Light_state = 1;
%        end    
%     elseif Speed_fb>=7 && Speed_fb<13
%        if Light_Distance<Stop_Dis_Low && Light_Distance>(Stop_Dis_Low-2)
%             Light_state = 1;
%        end 
%     elseif Speed_fb<7
%         if Light_Distance<(Stop_Dis_Low-5) && Light_Distance>(Stop_Dis_Low-6)
%             Light_state = 1;
%        end 
%     end
% elseif Phase == 2 || Phase == -1
%         Light_state = 0;
% end


if Phase ==1 || Phase ==3
    if Light_Distance< Stop_Distance && Light_Distance>(Stop_Distance-1)
        Light_state = 1;
    end
elseif Phase == 2 || Phase == 0
        Light_state = 0;
end

if Drive_start ==1
    Light_state = 0;
end
Light_flag = Light_state;

%%%%%%%%%%%%%%%%%%%%%%%%%%%%%%%%%%%%%%%%%%%%%%%%%%%%%%%%%%%%%%%%%%%%%%%%%%%
%  Prevent bus from accelerating and pass the stop flag trigger zone
if SLAM_seg_id_near>=277 && SLAM_seg_id_near<278 && (Phase ==1 || Phase ==3)
    Light_zone = 1;
else
    Light_zone = 0;
end
Light_acc = Light_zone;

== matlab function bus_roadtest_v3/Speed_profile/High level controller/SpeedProfile ==
  settings: updateMethod=DISCRETE
  data: Light_zone input; Stop_zone input; Deceleration_cons input; Acceleration_cons input; Idle_flag input; AEB_flag input; Light_flag input; Uturn_flag input; Slow_flag input; overtake_flag input; Delta_t input; Speed_fb input; Uturn_speed input; Speed_cmd output; Speed_desire output; Speed_set input; PPGF_Stop input; ACC_cmd input
    function [Speed_cmd, Speed_desire] = fcn(Light_zone, Stop_zone, Deceleration_cons, Acceleration_cons, Idle_flag, AEB_flag, Light_flag, Uturn_flag, Slow_flag, overtake_flag, Delta_t, Speed_fb, Uturn_speed, Speed_set,PPGF_Stop, ACC_cmd)



% PP_info = [Digital_gate, Believe_index];
% Pevent bus from passing the stops or lights

if (Light_zone==1 || Stop_zone==1) && Speed_fb>5
    Acceleration_cons = 0;
end
%%%%%%%%%%%%%%%%%%%%%%%%%%%%%%%%%%%%%%%%%%%%%%%%%%%%%%%%%%%%%%%%%%%%%%%%%%%
% Decide desired speed km/hr in descendinh order
Speed_desire = Speed_set;

if Slow_flag == 1
    Speed_desire = min(Speed_desire,10);
end

if Uturn_flag == 1
    Speed_desire = min(Speed_desire,Uturn_speed);
end

if overtake_flag == 1
    Speed_desire = min(Speed_desire,5);
end

if PPGF_Stop ==1
    Speed_desire = min(Speed_desire,5);
end

if Light_flag ==1
    Speed_desire = 0;
end

if Idle_flag ==1
    Speed_desire = 0;
end

%%%%%%%%%%%%%%%%%%%%%%%%%%%%%%%%%%%%%%%%%%%%%%%%%%%%%%%%%%%%%%%%%%%%%%%%%%%
%This part is for handling Idle flag
%km/h 2 m/s
Speed_fb = Speed_fb/3.6;
Speed_desire = Speed_desire/3.6;

if (Speed_fb > Speed_desire)
    Speed_cmd = Speed_fb - Deceleration_cons*Delta_t;
    if Speed_cmd<0
        Speed_cmd = 0;    
    end
elseif (Speed_fb < Speed_desire)
    Speed_cmd = Speed_fb + Acceleration_cons*Delta_t;
    if Speed_cmd>Speed_desire
        Speed_cmd = Speed_desire;
    end
else
    Speed_cmd = Speed_desire;
end

%m/s 2 km/h
Speed_cmd  = Speed_cmd *3.6;
Speed_desire = Speed_desire*3.6;
Speed_cmd = min(Speed_cmd,ACC_cmd);
%%%%%%%%%%%%%%%%%%%%%%%%%%%%%%%%%%%%%%%%%%%%%%%%%%%%%%%%%%%%%%%%%%%%%%%%%%%
if AEB_flag==1
    Speed_cmd = 0;  
end
%%%%%%%%%%%%%%%%%%%%%%%%%%%%%%%%%%%%%%%%%%%%%%%%%%%%%%%%%%%%%%%%%%%%%%%%%%%

== matlab function bus_roadtest_v3/Target_planner/Enabled Subsystem/Dijkstra ==
  data: nodes input; dist output; segments input; start_id input; finish_id input; path_2 output size=length(nodes(:,1)); nn output
function [dist,path_2,nn] = dijkstra(nodes,segments,start_id,finish_id)

node_ids = nodes(:,1);
[num_map_pts,cols] = size(nodes);
table = zeros(num_map_pts,2);%sparse(num_map_pts,2);
shortest_distance = Inf(num_map_pts,1);
settled = zeros(num_map_pts,1);
path = zeros(num_map_pts,num_map_pts);
col = 2;
pidx = find(start_id == node_ids);
shortest_distance(pidx(1)) = 0;
table(pidx(1),col) = 0;
settled(pidx(1)) = 1;
path(pidx(1),1) = start_id;
zz = find(finish_id == node_ids);

while settled(zz(1)) == 0
    % update the table
    table(:,col-1) = table(:,col);
    table(pidx(1),col) = 0;
    % find neighboring nodes in the segments list
    neighbor_ids = segments(node_ids(pidx(1)) == segments(:,2),3);
    % calculate the distances to the neighboring nodes and keep track of the paths
    for k = 1:length(neighbor_ids)
        cidx = find(neighbor_ids(k) == node_ids);
        if ~settled(cidx(1))
            d = sqrt(sum((nodes(pidx(1),2:cols) - nodes(cidx(1),2:cols)).^2));
            if (table(cidx(1),col-1) == 0) || (table(cidx(1),col-1) > (table(pidx(1),col-1) + d))
                table(cidx(1),col) = table(pidx(1),col-1) + d;
                path_nozero_index = find(path(pidx(1),:) ~= 0 );
                tmp_path = zeros(1,length(path_nozero_index));
                for m = 1 : length(path_nozero_index)
                    tmp_path(m) = path(pidx(1),path_nozero_index(m));
                end
                path(cidx(1),1:m+1) = [tmp_path neighbor_ids(k)];
            else
                table(cidx(1),col) = table(cidx(1),col-1);
            end
        end
    end
    % find the minimum non-zero value in the table and save it
    nidx = find(table(:,col));
    ndx = find(table(nidx,col) == min(table(nidx,col)));
    if isempty(ndx)
        break;
    else
        pidx = nidx(ndx(1));
        shortest_distance(pidx) = table(pidx,col);
        settled(pidx) = 1;
    end
end

dist = shortest_distance(zz(1));
nn = length(find(path(zz(1),:)~=0));
path_1 = path(zz(1),1:nn);
path_2 = path_1';

== matlab function bus_roadtest_v3/Target_planner/EndPointDecision ==
  data: Vehicle_state input; End_x output; Path_x_0 input size=length(nodes(:,1)); Path_y_0 input size=length(nodes(:,1)); forward_length input; End_y output; path_length output
function [End_x,End_y,path_length] = EndPointDecision(Vehicle_state,Path_x_0,Path_y_0,forward_length)

x = Vehicle_state(1,1); %vehicle global coordinate
y = Vehicle_state(2,1);

Path_x = Path_x_0;
Path_y = Path_y_0;

%% Target plan
Path_RES_0 = zeros(20000,2);
Path_RES_0_1 = zeros(20000,2);
Res = 0.1;
count = 0;
count_1 = 0;
break_count = 0;
target_k = floor(forward_length/Res);

%找出切成10公分之投影點
Length_1 = ((Path_x(2)-Path_x(1))^2+(Path_y(2)-Path_y(1))^2)^0.5;
ang_1 = atan2(Path_y(2)-Path_y(1),Path_x(2)-Path_x(1));
if Length_1 > Res
    for j = 1:round(Length_1/Res)
        Path_RES_0_1(j,1) = Path_x(1) + (j-1)*Res*cos(ang_1);
        Path_RES_0_1(j,2) = Path_y(1) + (j-1)*Res*sin(ang_1);
        count_1 = j;
    end
else
    Path_RES_0_1(1,1) = Path_x(1);
    Path_RES_0_1(1,2) = Path_y(1);
    count_1 = 1;
end
Path_RES_1 = Path_RES_0_1((1:count_1),:);
ob_distance = (x-Path_RES_1(:,1)).^2 + (y - Path_RES_1(:,2)).^2;
[none,v_i] = min(ob_distance);
x_ob = Path_RES_1(v_i,1);
y_ob = Path_RES_1(v_i,2);
o_i = count_1-v_i;

if numel(Path_x(:,1))-2 >=1
    for i = 1:numel(Path_x(:,1))-2
        k = i+1;
        if break_count == 0
            Length = ((Path_x(k+1)-Path_x(k))^2+(Path_y(k+1)-Path_y(k))^2)^0.5;
            ang = atan2(Path_y(k+1)-Path_y(k),Path_x(k+1)-Path_x(k));
            if Length >= Res
                index_j = round(Length/Res);
                for j = 1:index_j
                    Path_RES_0(j+count,1) = Path_x(k) + (j-1)*Res*cos(ang);
                    Path_RES_0(j+count,2) = Path_y(k) + (j-1)*Res*sin(ang);
                end
                count = count + index_j;
%                 clear index_j;
            else
                Path_RES_0(1+count,1) = Path_x(k);
                Path_RES_0(1+count,2) = Path_y(k);
                count = count + 1;
            end
            if count > target_k - o_i
                break_count = 1;
            end
            target_forward_i = k;
        end
    end
else
    Path_RES_0 = [];
    count = 0;
end

temp = target_k+v_i;
if isempty(Path_RES_0) == 1
    if temp <= length(Path_RES_1(:,1))
        Path_RES = Path_RES_1(v_i:temp,:);
        End_x = Path_RES(target_k,1);% global
        End_y = Path_RES(target_k,2);
        case_1 = 1;
        path_length = target_k*0.1;
    else
        Path_RES = Path_RES_1(v_i:end,:);
        End_x = Path_RES(end,1);% global
        End_y = Path_RES(end,2);
        case_1 = 2;
        path_length = length(Path_RES)*0.1;
    end
else
    Path_RES = [Path_RES_1(v_i:end,:);Path_RES_0((1:count),:)];
    if target_k-o_i <= count
        End_x = Path_RES(target_k,1);% global
        End_y = Path_RES(target_k,2);
        case_1 = 3;
        path_length = target_k*0.1;
    else
        End_x = Path_RES(count+o_i,1);% global
        End_y = Path_RES(count+o_i,2);
        case_1 = 4;
        path_length = (count+o_i)*0.1;
    end
end
